simulink subsystem "Ec_Diferencial"  (R2023b)
settings: Solver=VariableStepAuto  StartTime=0.0  StopTime=10.0  RelTol=1e-3
undefined symbols (not defined in the file): B, J, km, L, R, Ra
settings Model: Creator=marqu  LastModifiedBy=marqu

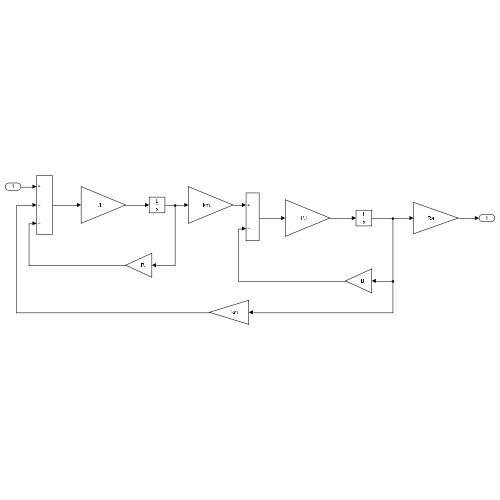
[thumbnail: Simulink's stored preview of the top-level diagram]
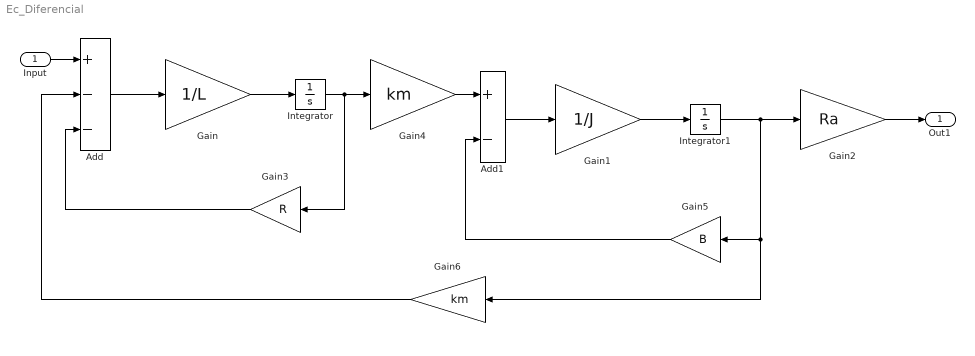
== system Ec_Diferencial ==
  Input : Inport
  Add : Sum  Inputs=+--
  Add1 : Sum  Inputs=+-
  Gain : Gain  Gain=1/L
  Gain1 : Gain  Gain=1/J
  Gain2 : Gain  Gain=Ra
  Gain3 : Gain  Gain=R
  Gain4 : Gain  Gain=km
  Gain5 : Gain  Gain=B
  Gain6 : Gain  Gain=km
  Integrator : Integrator
  Integrator1 : Integrator
  Out1 : Outport
  wires:
  Gain5/1 -> Add1/2
  Gain3/1 -> Add/3
  Add/1 -> Gain/1
  Gain1/1 -> Integrator1/1
  Add1/1 -> Gain1/1
  Gain6/1 -> Add/2
  Gain4/1 -> Add1/1
  Integrator1/1 -> Gain6/1, Gain5/1, Gain2/1
  Integrator/1 -> Gain3/1, Gain4/1
  Gain/1 -> Integrator/1
  Input/1 -> Add/1
  Gain2/1 -> Out1/1
